simulink model "m"  (R2026a)
settings: Solver=VariableStepAuto  StopTime=1.0
values from neighbouring files (symbols this model uses):
  b = 0.1    [simulation_data.mat]
  J = 0.01    [simulation_data.mat]
  K = 0.01    [simulation_data.mat]
  L = 0.5    [simulation_data.mat]
  R = 1    [simulation_data.mat]
libraries: simulink x1
settings Model: Creator=Nikhil  LastModifiedBy=Nikhil

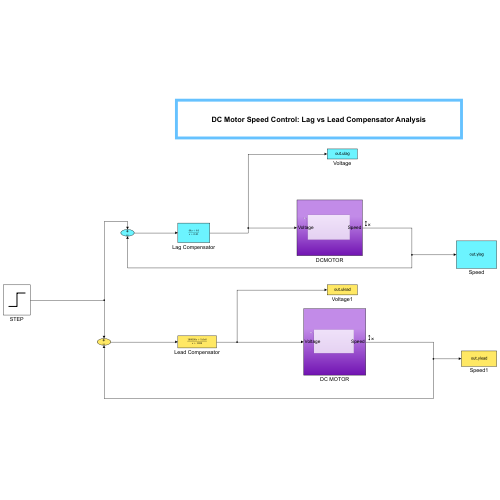
[thumbnail: Simulink's stored preview of the top-level diagram]
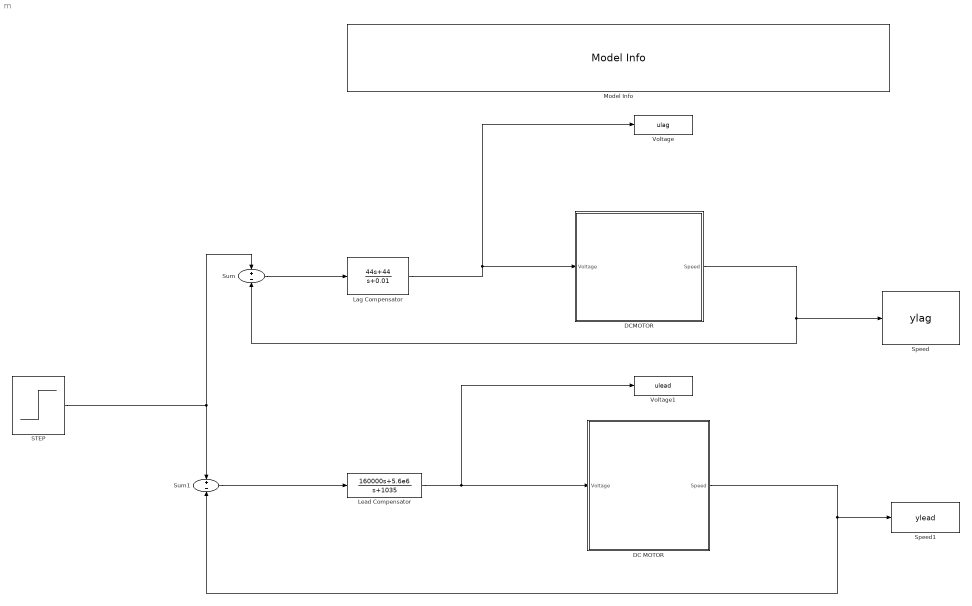
== system m ==
  DC MOTOR : Subsystem
  DCMOTOR : Subsystem
  Lag Compensator : TransferFcn  Numerator=[44 44]  Denominator=[1 0.01]
  Lead Compensator : TransferFcn  Numerator=[160000 5.6e6]  Denominator=[1 1035]
  Model Info : simulink/Model-Wide Utilities/Model Info  Frame=off  DisplayStringWithTags=DC Motor Speed Control: Lag vs Lead Compensator Analysis  HorizontalTextAlignment=Center  LeftAlignmentValue=0.5
  STEP : Step  Time=0  SampleTime=0
  Speed : ToWorkspace  VariableName=ylag  SampleTime=-1
  Speed1 : ToWorkspace  VariableName=ylead  SampleTime=-1
  Sum : Sum  Inputs=+-
  Sum1 : Sum  Inputs=+-
  Voltage : ToWorkspace  VariableName=ulag  SampleTime=-1
  Voltage1 : ToWorkspace  VariableName=ulead  SampleTime=-1
  wires:
  DCMOTOR/1(Speed) -> Speed/1, Sum/2
  Sum/1 -> Lag Compensator/1
  Lag Compensator/1 -> Voltage/1, DCMOTOR/1(Voltage)
  Sum1/1 -> Lead Compensator/1
  DC MOTOR/1(Speed) -> Sum1/2, Speed1/1
  STEP/1 -> Sum/1, Sum1/1
  Lead Compensator/1 -> DC MOTOR/1(Voltage), Voltage1/1

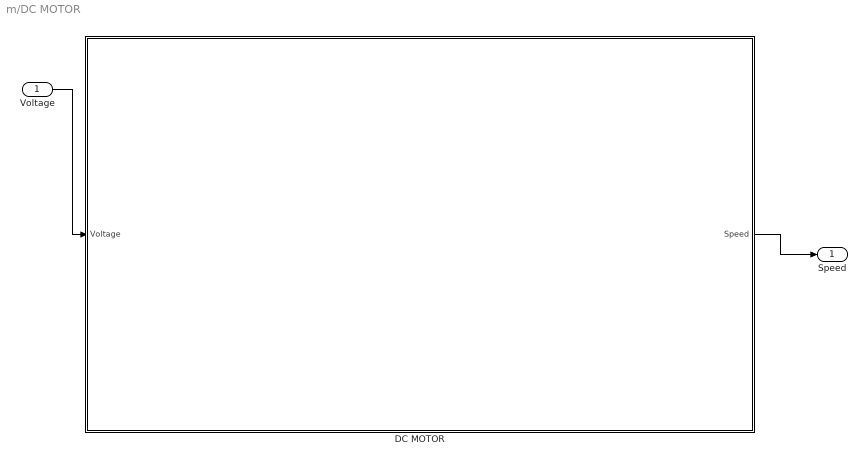
== system m/DC MOTOR ==
  Voltage : Inport
  DC MOTOR : Subsystem
  Speed : Outport
  wires:
  Voltage/1 -> DC MOTOR/1(Voltage)
  DC MOTOR/1(Speed) -> Speed/1

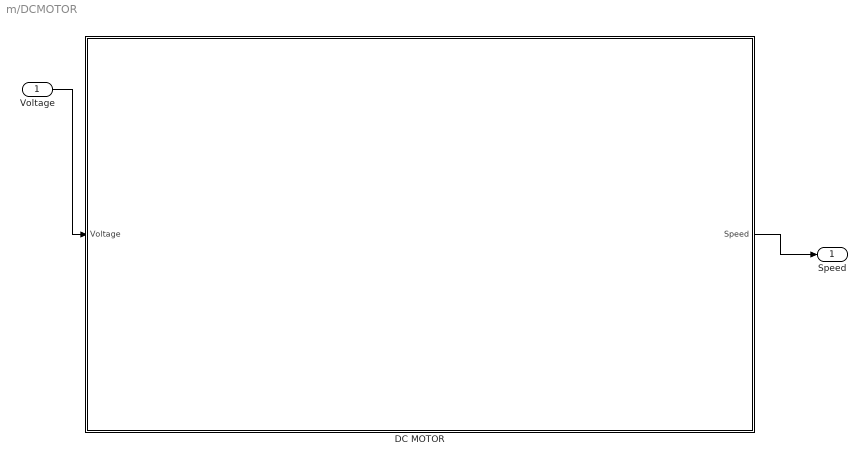
== system m/DCMOTOR ==
  Voltage : Inport
  DC MOTOR : Subsystem
  Speed : Outport
  wires:
  Voltage/1 -> DC MOTOR/1(Voltage)
  DC MOTOR/1(Speed) -> Speed/1

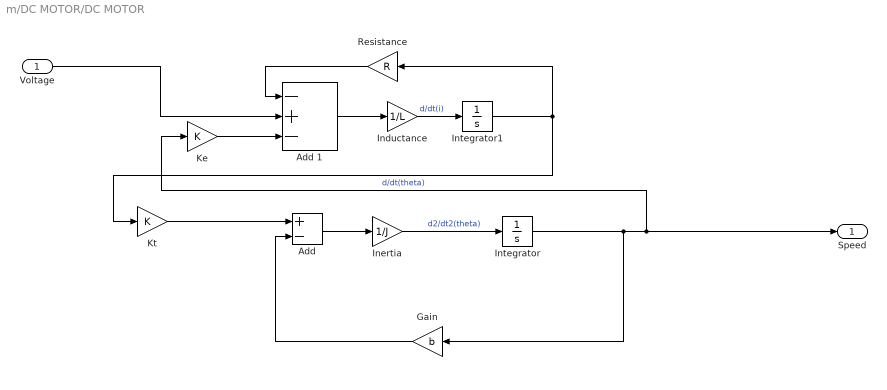
== system m/DC MOTOR/DC MOTOR ==
  Voltage : Inport
  Add : Sum  Inputs=+-
  Add 1 : Sum  Inputs=-+-
  Gain : Gain  Gain=b
  Inductance : Gain  Gain=1/L
  Inertia : Gain  Gain=1/J
  Integrator : Integrator
  Integrator1 : Integrator
  Ke : Gain  Gain=K
  Kt : Gain  Gain=K
  Resistance : Gain  Gain=R
  Speed : Outport
  wires:
  Resistance/1 -> Add 1/1
  Add/1 -> Inertia/1
  Inductance/1 -> Integrator1/1  "d/dt(i)"
  Integrator1/1 -> Resistance/1, Kt/1
  Integrator/1 -> Gain/1, Speed/1, Ke/1  "d/dt(theta)"
  Ke/1 -> Add 1/3
  Gain/1 -> Add/2
  Kt/1 -> Add/1
  Add 1/1 -> Inductance/1
  Inertia/1 -> Integrator/1  "d2/dt2(theta)"
  Voltage/1 -> Add 1/2

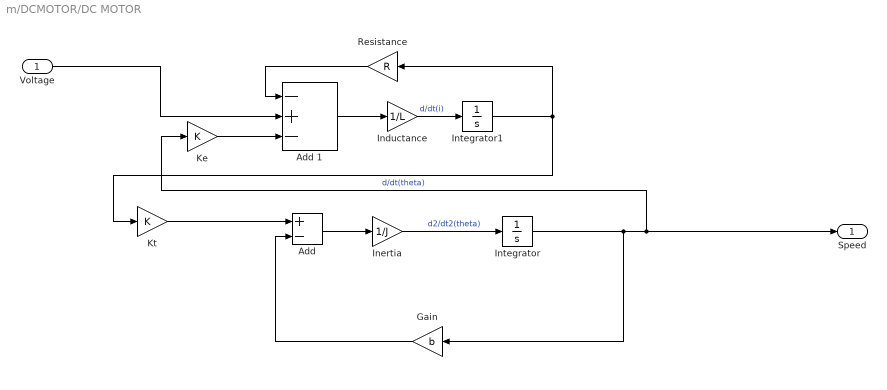
== system m/DCMOTOR/DC MOTOR ==
  Voltage : Inport
  Add : Sum  Inputs=+-
  Add 1 : Sum  Inputs=-+-
  Gain : Gain  Gain=b
  Inductance : Gain  Gain=1/L
  Inertia : Gain  Gain=1/J
  Integrator : Integrator
  Integrator1 : Integrator
  Ke : Gain  Gain=K
  Kt : Gain  Gain=K
  Resistance : Gain  Gain=R
  Speed : Outport
  wires:
  Resistance/1 -> Add 1/1
  Add/1 -> Inertia/1
  Inductance/1 -> Integrator1/1  "d/dt(i)"
  Integrator1/1 -> Resistance/1, Kt/1
  Integrator/1 -> Gain/1, Speed/1, Ke/1  "d/dt(theta)"
  Ke/1 -> Add 1/3
  Gain/1 -> Add/2
  Kt/1 -> Add/1
  Add 1/1 -> Inductance/1
  Inertia/1 -> Integrator/1  "d2/dt2(theta)"
  Voltage/1 -> Add 1/2
